simulink model "es_tipo_esame_3_schema"  (R2021b)
settings: Solver=VariableStepAuto  StartTime=0.0  StopTime=20.0  RelTol=1e-3
values from neighbouring files (symbols this model uses):
  Tp = 1    [es_tipo_esame_3.m]
libraries: cstblocks x6
settings Model: Creator=francescafornasier  LastModifiedBy=francescafornasier

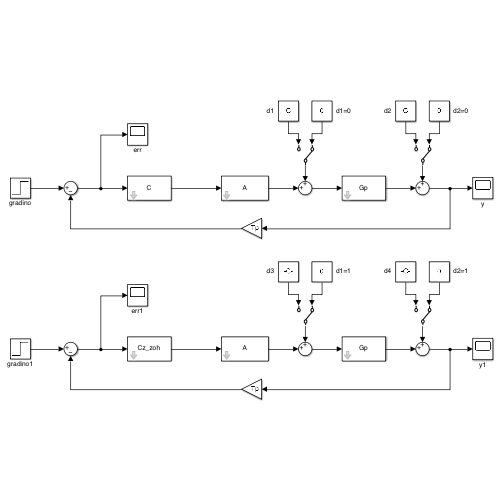
[thumbnail: Simulink's stored preview of the top-level diagram]
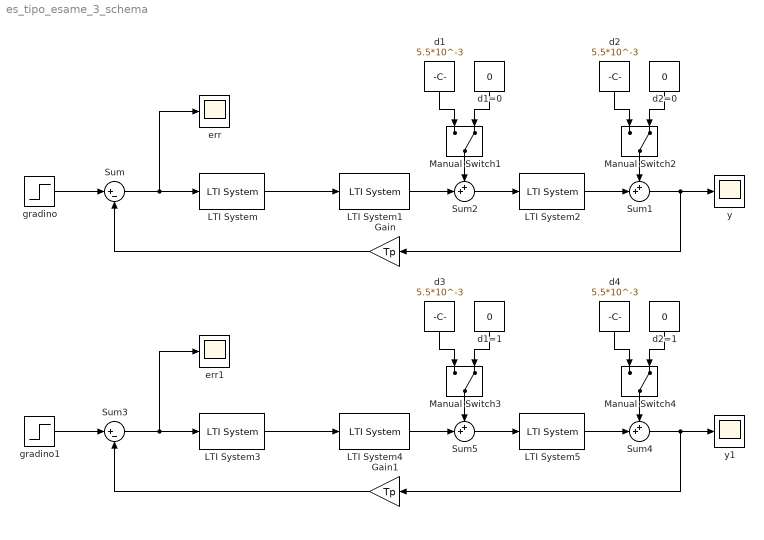
== system es_tipo_esame_3_schema ==
  Gain : Gain  Gain=Tp
  Gain1 : Gain  Gain=Tp
  LTI System : cstblocks/LTI System  sys=C  IC=[]
  LTI System1 : cstblocks/LTI System  sys=A  IC=[]
  LTI System2 : cstblocks/LTI System  sys=Gp  IC=[]
  LTI System3 : cstblocks/LTI System  sys=Cz_zoh  IC=[]
  LTI System4 : cstblocks/LTI System  sys=A  IC=[]
  LTI System5 : cstblocks/LTI System  sys=Gp  IC=[]
  Manual Switch{1..4} (4 alike) : ManualSwitch  CurrentSetting=0
  Sum : Sum  Inputs=|+-
  Sum{1..2,4..5} (4 alike) : Sum  Inputs=++|
  Sum3 : Sum  Inputs=|+-
  d{1..4} (4 alike) : Constant  Value=5.5*10^-3
  d1=0 : Constant  Value=0
  d1=1 : Constant  Value=0
  d2=0 : Constant  Value=0
  d2=1 : Constant  Value=0
  err : Scope
  err1 : Scope
  gradino : Step  Time=0  SampleTime=0
  gradino1 : Step  Time=0  SampleTime=0
  y : Scope
  y1 : Scope
  wires:
  Manual Switch2/1 -> Sum1/1
  d1/1 -> Manual Switch1/1
  d1=0/1 -> Manual Switch1/2
  Manual Switch1/1 -> Sum2/1
  gradino/1 -> Sum/1
  Sum/1 -> err/1, LTI System/1
  LTI System1/1 -> Sum2/2
  d2=0/1 -> Manual Switch2/2
  LTI System/1 -> LTI System1/1
  d2/1 -> Manual Switch2/1
  Sum1/1 -> y/1, Gain/1
  LTI System2/1 -> Sum1/2
  Sum2/1 -> LTI System2/1
  Gain/1 -> Sum/2
  d3/1 -> Manual Switch3/1
  gradino1/1 -> Sum3/1
  d4/1 -> Manual Switch4/1
  Sum4/1 -> y1/1, Gain1/1
  Manual Switch3/1 -> Sum5/1
  Sum5/1 -> LTI System5/1
  Manual Switch4/1 -> Sum4/1
  LTI System3/1 -> LTI System4/1
  LTI System5/1 -> Sum4/2
  d2=1/1 -> Manual Switch4/2
  LTI System4/1 -> Sum5/2
  d1=1/1 -> Manual Switch3/2
  Sum3/1 -> err1/1, LTI System3/1
  Gain1/1 -> Sum3/2
